simulink model "Controller_First_Test_new"  (R2019b)
settings: Solver=VariableStepAuto  StartTime=0.0  StopTime=1000  RelTol=1e-3
undefined symbols (not defined in the file or in its folder): A, B, C, Continuous, D, K, K_u, Time
libraries: ctrlSharedLib x1, realtime_pacer_lib x1, simulink x1
settings Model: Creator=Presentatie  LastModifiedBy=Presentatie

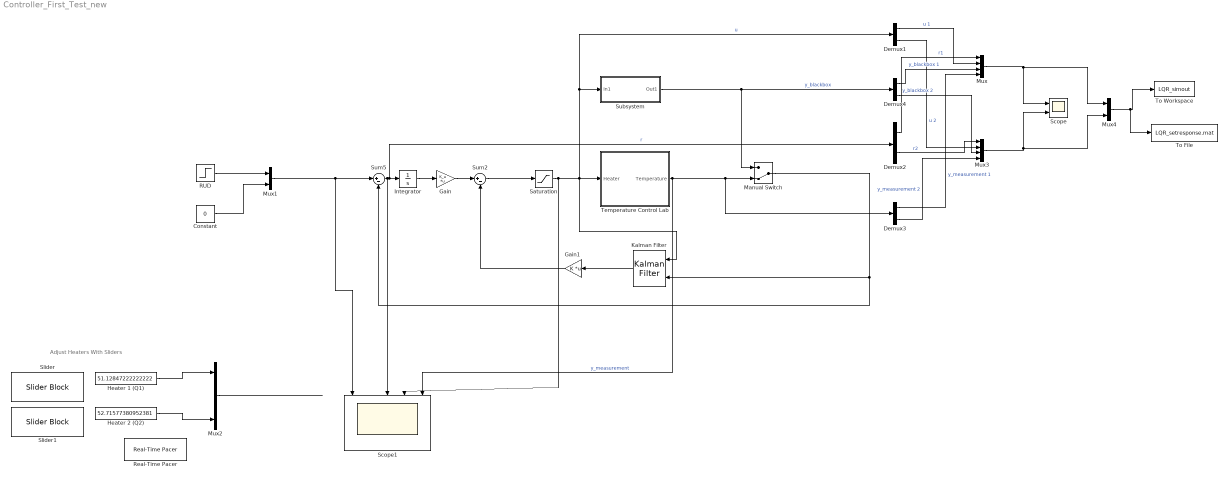
== system Controller_First_Test_new ==
  note: Adjust Heaters With Sliders
  Constant : Constant  Value=0
  Demux{1..4} (4 alike) : Demux  Outputs=2
  Gain : Gain  Gain=K_u  Multiplication=Matrix(K*u)
  Gain1 : Gain  Gain=K  Multiplication=Matrix(K*u)
  Heater 1 (Q1) : Constant  Value=51.12847222222222
  Heater 2 (Q2) : Constant  Value=52.71577380952381
  Integrator : Integrator
  Kalman Filter : ctrlSharedLib/Kalman Filter  TimeDomain=Continuous-Time  UseCurrentEstimator=on  ModelSource=Individual A, B, C, D matrices  ModelSourceVariable=ss(0.95,1,1,0,1)  A=A  B=B  C=C  D=D  NumberOfStates=1  NumberOfInputs=1  NumberOfOutputs=1  InitialEstimateSource=Dialog  X0=0  P0=10  UseK=off  UseGH=off  NumberOfProcessNoiseInputs=1  G=1  TimeInvariantG=on  H=0  TimeInvariantH=on  Q=0.05  TimeInvariantQ=on  R=1  TimeInvariantR=on  N=0  TimeInvariantN=on  AddInputPort=on  AddEnablePort=off  OutputEstimatedY=off  OutputP=off  Ts=-1
      settings: SourceProductBaseCode=CT
  Manual Switch : ManualSwitch  CurrentSetting=0
  Mux : Mux
  Mux1 : Mux  Inputs=2
  Mux2 : Mux  Inputs=3
  Mux3 : Mux
  Mux4 : Mux  Inputs=2
  "RUD " : Step  Time=30  After=50  SampleTime=0
  Real-Time Pacer : realtime_pacer_lib/Real-Time Pacer  simTimePerRealTime=1
  Saturation : Saturate
  Scope : Scope  NumInputPorts=2
  Scope1 : Scope  NumInputPorts=5
  Slider : SliderBlock  TickInterval=20
  Slider1 : SliderBlock  TickInterval=20
  Subsystem : Subsystem
  Sum2 : Sum  Inputs=|+-
  Sum5 : Sum  Inputs=|+-
  Temperature Control Lab : Subsystem
      mask Display: image('tclab.png');
  To File : ToFile  Filename=LQR_setresponse.mat  SaveFormat=Timeseries
  To Workspace : ToWorkspace  VariableName=LQR_simout  SaveFormat=Timeseries  SampleTime=-1
  wires:
  Mux/1 -> Mux4/1, Scope/1
  "RUD "/1 -> Mux1/1
  Constant/1 -> Mux1/2
  Heater 2 (Q2)/1 -> Mux2/3
  Mux2/1 -> ?
  Heater 1 (Q1)/1 -> Mux2/1
  Mux1/1 -> Sum5/1, Scope1/1
  Integrator/1 -> Gain/1
  Gain/1 -> Sum2/1
  Gain1/1 -> Sum2/2
  Sum2/1 -> Saturation/1
  Kalman Filter/1 -> Gain1/1
  Saturation/1 -> Subsystem/1(In1), Demux1/1, Kalman Filter/1, Temperature Control Lab/1(Heater), Scope1/4  "u"
  Sum5/1 -> Integrator/1, Demux2/1, Scope1/3  "r"
  Manual Switch/1 -> Kalman Filter/2, Sum5/2
  Temperature Control Lab/1(Temperature) -> Demux3/1, Manual Switch/2, Scope1/5  "y_measurement"
  Subsystem/1(Out1) -> Manual Switch/1, Demux4/1  "y_blackbox"
  Demux2/1 -> Mux/1  "r1"
  Demux1/1 -> Mux/2  "u 1"
  Demux4/1 -> Mux/3  "y_blackbox 1"
  Demux3/1 -> Mux/4  "y_measurement 1"
  Demux2/2 -> Mux3/1  "r2"
  Demux1/2 -> Mux3/2  "u 2"
  Demux4/2 -> Mux3/3  "y_blackbox 2"
  Demux3/2 -> Mux3/4  "y_measurement 2"
  Mux3/1 -> Mux4/2, Scope/2
  Mux4/1 -> To Workspace/1, To File/1

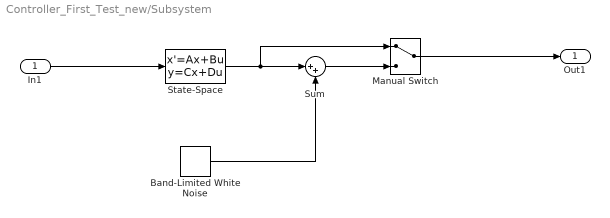
== system Controller_First_Test_new/Subsystem ==
  In1 : Inport
  Band-Limited White Noise : simulink/Sources/Band-Limited White Noise  Cov=[0.1]  Ts=0.1  seed=[23341]
  Manual Switch : ManualSwitch
  State-Space : StateSpace  A=A  B=B  C=C  D=D  InitialCondition=0
  Sum : Sum  Inputs=|++
  Out1 : Outport
  wires:
  In1/1 -> State-Space/1
  Band-Limited White Noise/1 -> Sum/2
  State-Space/1 -> Manual Switch/1, Sum/1
  Sum/1 -> Manual Switch/2
  Manual Switch/1 -> Out1/1

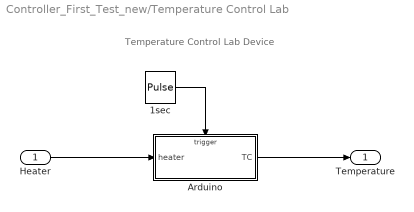
== system Controller_First_Test_new/Temperature Control Lab ==
  note: Temperature Control Lab Device
  Heater : Inport
  1sec : DiscretePulseGenerator  PulseType=Time based  Period=1  PulseWidth=50
  Arduino : Subsystem  TreatAsAtomicUnit=on
  Temperature : Outport  VectorParamsAs1DForOutWhenUnconnected=off
  wires:
  1sec/1 -> Arduino/Trigger
  Arduino/1(TC) -> Temperature/1
  Heater/1 -> Arduino/1(heater)

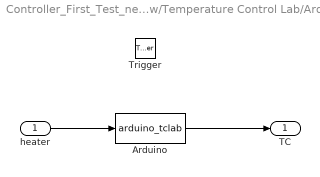
== system Controller_First_Test_new/Temperature Control Lab/Arduino ==
  heater : Inport  LatchByDelayingOutsideSignal=on
  Trigger : TriggerPort  VariantControl=Variant
  Arduino : MATLABFcn  MATLABFcn=arduino_tclab
  TC : Outport  InitialOutput=[23 23]  VectorParamsAs1DForOutWhenUnconnected=off
  wires:
  heater/1 -> Arduino/1
  Arduino/1 -> TC/1
